simulink model "sensor_fusion_2"  (R2022b)
settings: Solver=FixedStepDiscrete  StartTime=0.0  StopTime=200  RelTol=1e-3  EnableMultiTasking=on
values from neighbouring files (symbols this model uses):
  A = [1.06559801427  0.0478097134081  -0.0142426631232; 0.0478097134081  0.959164863261  -0.0359507847494; -0.0142426631232  -0.0359507847494  0.982079248423]    [run1.mat]    (also in run2.mat)
  b = [2.14306210308 15.720848335 -0.863601368467]    [run1.mat]    (also in run2.mat)
  lut_in_model = [0.705252988187 2.8039042404 3.65243764674 4.31474263379 6.41199264306 8.27776188122 9.84362520272 10.5320461641 11.7803083612 12.6369678359 13.2471074191 13.768187271 ... (20 elements, 1x20)]    [lut5.mat]    (also in run1.mat; run2.mat)
  lut_out_model = [3.92727272727 4.14545454545 4.36363636364 4.58181818182 5.45454545455 6.54545454545 7.63636363636 8.72727272727 9.81818181818 10.9090909091 12 13.0909090909 ... (20 elements, 1x20)]    [lut5.mat]    (also in run1.mat; run2.mat)
undefined symbols (not defined in the file or in its folder): Discrete, ODR, Time
libraries: raspberrypiBasiclib x6, raspberrypiIMUsensorslib x2, matrix_library x1, ctrlSharedLib x1, dspsigops x1, raspberrypiAVlib x1, slpidlib x1
settings Model: Creator=sjohnson  LastModifiedBy=sjohnson
settings SolverCC: PositivePriorityOrder=on
settings OptimizationCC: EnhancedBackFolding=on  PassReuseOutputArgsAs=Individual arguments  ZeroExternalMemoryAtStartup=off  ZeroInternalMemoryAtStartup=off  MaxStackSize=64  OptimizeBlockOrder=speed  DifferentSizesBufferReuse=on  OptimizationCustomize=off  EfficientTunableParamExpr=on
settings DebuggingCC: ParameterTunabilityLossMsg=error
settings HardwareCC: ProdBitPerPointer=32  ProdBitPerSizeT=32  ProdBitPerPtrDiffT=32  ProdLargestAtomicInteger=Long  ProdLargestAtomicFloat=Double  ProdWordSize=32  ProdLongLongMode=on  ProdHWDeviceType=ARM Compatible->ARM Cortex  UseEmbeddedCoderFeatures=off  UseSimulinkCoderFeatures=off
settings RTWCC: Description=Embedded Coder  SystemTargetFile=ert.tlc  HardwareBoard=Raspberry Pi  TLCOptions="-aInlineSetEventsForThisBaseRateFcn=TLC_FALSE -aSuppressMultiTaskScheduler=TLC_FALSE  -aRateBasedStepFcn=0"  TemplateMakefile=ert_default_tmf  Toolchain=GNU GCC Embedded Linux  BuildConfiguration=Faster Runs
settings CodeAppCC: ForceParamTrailComments=on  IgnoreCustomStorageClasses=off  OperatorAnnotations=on  SimulinkDataObjDesc=on  SFDataObjDesc=on  InsertBlockDesc=on
settings ERTTargetCC: SupportNonInlinedSFcns=on  SupportVariableSizeSignals=on  ExtModeTransport=2  ExtModeStaticAlloc=on  ExtModeMexFile=ext_xcp  ExtModeIntrfLevel=Level2 - Open

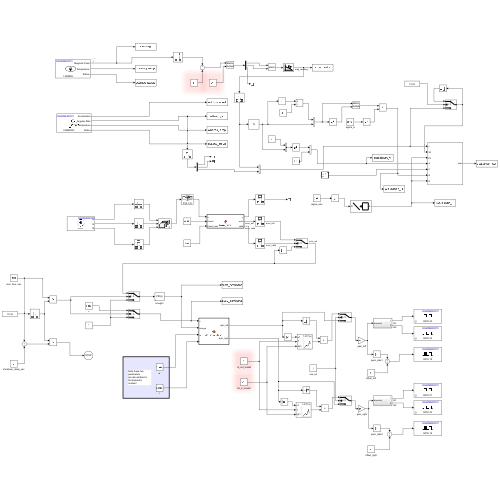
[thumbnail: Simulink's stored preview of the top-level diagram]
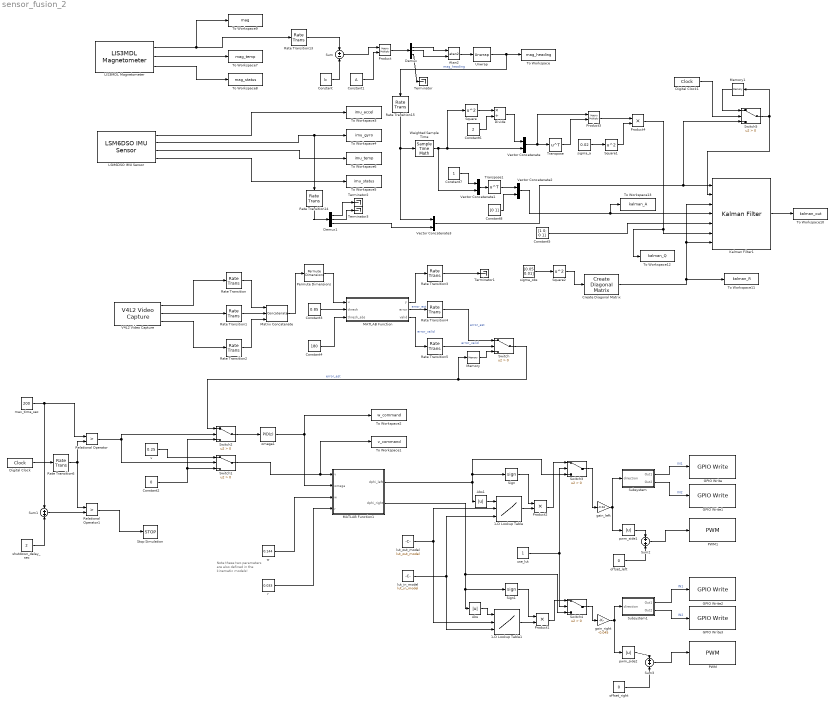
== system sensor_fusion_2 ==
  note: Note these two parameters
      | are also defined in the kinematic
      | models!
  1-D Lookup Table : Lookup_n-D  NumberOfTableDimensions=1  BreakpointsForDimension1Source=Input port  BreakpointsForDimension1=[-5:5]  IndexSearchMethod=Linear search  TableSource=Input port  Table=tanh([-5:5])  InterpMethod=Cubic spline  InternalRulePriority=Speed  RndMeth=Simplest
      settings: InputPortMap=u0,p221,p5
  1-D Lookup Table1 : Lookup_n-D  NumberOfTableDimensions=1  BreakpointsForDimension1Source=Input port  BreakpointsForDimension1=[-5:5]  IndexSearchMethod=Linear search  TableSource=Input port  Table=tanh([-5:5])  InterpMethod=Cubic spline  InternalRulePriority=Speed  RndMeth=Simplest
      settings: InputPortMap=u0,p221,p5
  Abs : Abs  SaturateOnIntegerOverflow=off
  Abs1 : Abs  SaturateOnIntegerOverflow=off
  Atan2 : Trigonometry  Operator=atan2
  Constant : Constant  Value=b  SampleTime=-1
  Constant1 : Constant  Value=A  SampleTime=-1
  Constant2 : Constant  Value=0
  Constant3 : Constant  Value=0.85
  Constant4 : Constant  Value=180
  Constant5 : Constant  Value=[1 0; 0 1]  SampleTime=-1
  Constant6 : Constant  Value=2  SampleTime=-1
  Constant7 : Constant  SampleTime=-1
  Constant8 : Constant  Value=[0 1]  VectorParams1D=off  SampleTime=-1
  Create Diagonal Matrix : matrix_library/Create Diagonal Matrix
      settings: LibrarySourceBlock=|
      | simulink/Matrix
      | Operations/Create Diagonal
      | Matrix
  Demux : Demux  Outputs=3
  Demux1 : Demux  Outputs=3
  Digital Clock : DigitalClock  SampleTime=1/30
  Digital Clock1 : DigitalClock  SampleTime=1/30
  Divide : Product  Inputs=*/
  GPIO Write : raspberrypiBasiclib/GPIO Write  board=Pi 4 Model B  gpio=23  direction=Output  blockPlatform=Raspberry Pi
  GPIO Write1 : raspberrypiBasiclib/GPIO Write  board=Pi 4 Model B  gpio=24  direction=Output  blockPlatform=Raspberry Pi
  GPIO Write2 : raspberrypiBasiclib/GPIO Write  board=Pi 4 Model B  gpio=27  direction=Output  blockPlatform=Raspberry Pi
  GPIO Write3 : raspberrypiBasiclib/GPIO Write  board=Pi 4 Model B  gpio=22  direction=Output  blockPlatform=Raspberry Pi
  Kalman Filter1 : ctrlSharedLib/Kalman Filter  TimeDomain=Discrete-Time  UseCurrentEstimator=on  ModelSource=Input port  ModelSourceVariable=ss(0.95,1,1,0,1)  A=0.95  B=1  C=1  D=0  NumberOfStates=2  NumberOfInputs=1  NumberOfOutputs=2  InitialEstimateSource=Input port  X0=0  P0=10  UseK=off  UseGH=off  NumberOfProcessNoiseInputs=1  G=1  TimeInvariantG=on  H=0  TimeInvariantH=on  Q=0.05  TimeInvariantQ=off  R=[0.0025 0; 0 0.0001]  TimeInvariantR=off  N=0  TimeInvariantN=on  AddInputPort=off  AddEnablePort=off  OutputEstimatedY=off  OutputP=off  Ts=-1
  LIS3MDL Magnetometer : raspberrypiIMUsensorslib/LIS3MDL Magnetometer  I2CModule=1  I2CAddress=0x1E  IsActiveMagnetometer=on  IsActiveTemperature=on  IsStatus=on  SampleTime=1/30  MagnetometerRange=+/- 400 uT  MagnetometerODR=40 Hz
  LSM6DSO IMU Sensor : raspberrypiIMUsensorslib/LSM6DSO IMU Sensor  I2CModule=1  I2CAddress=0x6B  IsActiveAcceleration=on  IsActiveAngularRate=on  IsActiveTemperature=on  IsActiveStatus=on  IsActiveTimeStamp=off  SampleTime=1/30  QueueSizeFactor=3  AccelerometerRange=+/- 2g  AccelerometerODR=52 Hz  AccelSelectCompositeFilter=No filter  AccelLPF2BW=ODR/4  AccelHPFBW=ODR/4  GyroscopeRange=1000 dps  GyroscopeODR=52 Hz  EnableGyroHPF=off  GyroHPFBW=0.016 Hz  EnableGyroLPF=off  GyroLPFBWMode=0
  MATLAB Function : MATLAB Function  TreatAsAtomicUnit=on
  MATLAB Function1 : MATLAB Function  TreatAsAtomicUnit=on
  Matrix Concatenate : Concatenate  NumInputs=3  Mode=Multidimensional array  ConcatenateDimension=3
  Memory : Memory
  Memory1 : Memory  InheritSampleTime=on
  PWM : raspberrypiBasiclib/PWM  board=Pi 4 Model B  Pin_=19  Frequency=40  blockPlatform=Raspberry Pi
  PWM1 : raspberrypiBasiclib/PWM  board=Pi 4 Model B  Pin_=18  Frequency=40  blockPlatform=Raspberry Pi
  Permute Dimensions : PermuteDimensions  Order=[2,1,3]
  Product : Product  Multiplication=Matrix(*)
  Product1 : Product
  Product2 : Product
  Product3 : Product  Multiplication=Matrix(*)
  Product4 : Product
  Rate Transition{,1..6,13} (8 alike) : RateTransition
  Rate Transition14 : RateTransition  OutPortSampleTime=1/30
  Rate Transition15 : RateTransition  OutPortSampleTime=1/30
  Relational Operator : RelationalOperator  Operator=>  OutDataTypeStr=boolean  RndMeth=Simplest  InputSameDT=off
  Relational Operator1 : RelationalOperator  Operator=>  OutDataTypeStr=boolean  RndMeth=Simplest  InputSameDT=off
  Sign : Signum
  Sign1 : Signum
  Square : Math  Operator=square
  Square1 : Math  Operator=square
  Square2 : Math  Operator=square
  Stop Simulation : Stop
  Subsystem : Subsystem
  Subsystem1 : Subsystem
  Sum : Sum  Inputs=+-
  Sum1 : Sum
  Sum2 : Sum
  Sum3 : Sum
  Switch{,1..5} (6 alike) : Switch  Criteria=u2 > Threshold  SaturateOnIntegerOverflow=off  InputSameDT=off
  Terminator{,1..3} (4 alike) : Terminator
  To Workspace : ToWorkspace  VariableName=mag_heading  SaveFormat=Structure With Time  SampleTime=-1
  To Workspace1 : ToWorkspace  VariableName=v_command  SaveFormat=Structure With Time  SampleTime=-1
  To Workspace10 : ToWorkspace  VariableName=kalman_out  SaveFormat=Structure With Time  SampleTime=-1
  To Workspace11 : ToWorkspace  VariableName=kalman_R  SaveFormat=Structure With Time  SampleTime=-1
  To Workspace12 : ToWorkspace  VariableName=kalman_Q  SaveFormat=Structure With Time  SampleTime=-1
  To Workspace13 : ToWorkspace  VariableName=kalman_A  SaveFormat=Structure With Time  SampleTime=-1
  To Workspace2 : ToWorkspace  VariableName=w_command  SaveFormat=Structure With Time  SampleTime=-1
  To Workspace3 : ToWorkspace  VariableName=imu_accel  SaveFormat=Structure With Time  SampleTime=-1
  To Workspace4 : ToWorkspace  VariableName=imu_gyro  SaveFormat=Structure With Time  SampleTime=-1
  To Workspace5 : ToWorkspace  VariableName=imu_status  SaveFormat=Structure With Time  SampleTime=-1
  To Workspace6 : ToWorkspace  VariableName=imu_temp  SaveFormat=Structure With Time  SampleTime=-1
  To Workspace7 : ToWorkspace  VariableName=mag_temp  SaveFormat=Structure With Time  SampleTime=-1
  To Workspace8 : ToWorkspace  VariableName=mag_status  SaveFormat=Structure With Time  SampleTime=-1
  To Workspace9 : ToWorkspace  VariableName=mag  SaveFormat=Structure With Time  SampleTime=-1
  Transpose : Math  Operator=transpose
  Transpose1 : Math  Operator=transpose
  Unwrap : dspsigops/Unwrap  tol=pi  InputProcessing=Columns as channels (frame based)  running=off
  V4L2 Video Capture : raspberrypiAVlib/V4L2 Video Capture  DeviceName=/dev/video0  Resolution=640x480  CustomResolution=[ 320, 240 ]  PixelFormat=RGB  SampleTime=1/30  pixelOrder=planar  simOutput=Colorbars  imSizeSelection=320x240  imSize=[640, 480]  roi=[0, 0, 640, 480]  m_devName='/dev/video0'  blockPlatform=LINUX  HorizontalFlip=off  VerticalFlip=off  Brightness=0.5  Saturation=0.5  Contrast=0.5  Sharpness=0.5  CameraPan=0  CameraTilt=0  CameraZoom=0.5  EnableManualFocus=off  ManualFocus=0.5
  Vector Concatenate : Concatenate  Mode=Multidimensional array
  Vector Concatenate1 : Concatenate
  Vector Concatenate2 : Concatenate  Mode=Multidimensional array
  Vector Concatenate3 : Concatenate  Mode=Multidimensional array
  Weighted Sample Time : SampleTimeMath  TsampMathOp=Ts Only  weightValue=1
  gain_left : Gain  Gain=-0.04
  gain_right : Gain  Gain=-0.045
  lut_in_model : Constant  Value=lut_in_model
  lut_out_model : Constant  Value=lut_out_model
  max_time_sec : Constant  Value=200
  offset_left : Constant  Value=0
  offset_right : Constant  Value=0
  omega1 : slpidlib/PID Controller  Controller=PID  Form=Parallel  TimeDomain=Discrete-time  UseExternalTs=off  SampleTime=-1  IntegratorMethod=Forward Euler  FilterMethod=Forward Euler  ControllerParametersSource=internal  P=-1.5  I=0  UseKiTs=off  D=0  N=100  UseFilter=on  TunerSelectOption=Transfer Function Based (PID Tuner App)  InitialConditionSource=internal  InitialConditionForIntegrator=0  InitialConditionForFilter=0  DifferentiatorICPrevScaledInput=0  ExternalReset=none  TrackingMode=off  Kt=1  LimitOutput=off  SatLimitsSource=internal  UpperSaturationLimit=inf  LowerSaturationLimit=-inf  LinearizeAsGain=off  AntiWindupMode=none  Kb=1  LimitIntegrator=off  UpperIntegratorSaturationLimit=inf  LowerIntegratorSaturationLimit=-inf  POutMin=[]  POutMax=[]  IOutMin=[]  IOutMax=[]  DOutMin=[]  DOutMax=[]  NOutMin=[]  NOutMax=[]  SumOutMin=[]  SumOutMax=[]  SaturationOutMin=[]  SaturationOutMax=[]  PParamMin=[]  PParamMax=[]  IParamMin=[]  IParamMax=[]  DParamMin=[]  DParamMax=[]  NParamMin=[]  NParamMax=[]  KbParamMin=[]  KbParamMax=[]  KtParamMin=[]  KtParamMax=[]  KbOutMin=[]  KbOutMax=[]  KtOutMin=[]  KtOutMax=[]  IntegratorOutMin=[]  IntegratorOutMax=[]  FilterOutMin=[]  FilterOutMax=[]  SumI1OutMin=[]  SumI1OutMax=[]  SumI2OutMin=[]  SumI2OutMax=[]  SumI3OutMin=[]  SumI3OutMax=[]  SumI4OutMin=[]  SumI4OutMax=[]  SumDOutMin=[]  SumDOutMax=[]  DifferentiatorOutMin=[]  DifferentiatorOutMax=[]  FilterDiffOutCoefMin=[]  FilterDiffOutCoefMax=[]  ReciprocalOutMin=[]  ReciprocalOutMax=[]  SumDenOutMin=[]  SumDenOutMax=[]  SumNumOutMin=[]  SumNumOutMax=[]  DivideOutMin=[]  DivideOutMax=[]  UdiffTsProdOutMin=[]  UdiffTsProdOutMax=[]  NTsProdOutMin=[]  NTsProdOutMax=[]  UintegralTsProdOutMin=[]  UintegralTsProdOutMax=[]  UngainTsProdOutMin=[]  UngainTsProdOutMax=[]  ClampingZeroOutDataTypeStr=Inherit: Inherit via back propagation  ClampingZeroOutMin=[]  ClampingZeroOutMax=[]  FilterDenConstantOutDataTypeStr=Inherit: Inherit via back propagation  FilterDenConstantOutMin=[]  FilterDenConstantOutMax=[]  PCopyOutDataTypeStr=Inherit: Inherit via back propagation  PCopyOutMin=[]  PCopyOutMax=[]  NCopyOutDataTypeStr=Inherit: Inherit via back propagation  NCopyOutMin=[]  NCopyOutMax=[]  IntegratorContinuousStateAttributes=''  IntegratorStateMustResolveToSignalObject=off  IntegratorRTWStateStorageClass=Auto  FilterContinuousStateAttributes=''  FilterStateMustResolveToSignalObject=off  FilterRTWStateStorageClass=Auto  ParallelPVariant=InternalParameters  IdealPVariant=Disabled  IVariant=InternalParameters  DVariant=InternalParameters  IntegratorVariant=Discrete  SatVariant=Disabled  AWVariant=Passthrough  PCopyVariant=Disabled  TRVariant=Disabled  FdbkBlocksVariant=Forward  IdealPFdbkVariant=Disabled  SatFdbkVariant=Disabled  DerivativeFilterVariant=ForwardEulerFilter  NVariant=InternalParameters  NCopyVariant=Disabled  FilterICVariant=InternalICsFilter  IntegratorICVariant=InternalICs  ExternalResetVariant=Disabled  TRSumVariant=Passthrough  SumFdbkVariant=Disabled  SumVariant=Sum_PID  TsampFilterVariant=InternalTs  TsampNgainVariant=Passthrough  TsampIntegralVariant=Passthrough  ExternalSaturationOutDataTypeStr=Inherit: Same as second input
      settings: LibrarySourceBlock=simulink/Discrete/Discrete PID Controller
  pwm_side1 : Abs  SaturateOnIntegerOverflow=off
  pwm_side2 : Abs  SaturateOnIntegerOverflow=off
  r : Constant  Value=0.033
  shutdown_delay_sec : Constant  Value=2
  sigma_a : Constant  Value=0.02  SampleTime=-1
  sigma_obs : Constant  Value=[0.05 0.01]  SampleTime=-1
  use_lut : Constant
  v : Constant  Value=0.25
  w : Constant  Value=0.144
  wires:
  LSM6DSO IMU Sensor/3 -> To Workspace6/1
  LIS3MDL Magnetometer/3 -> To Workspace8/1
  LSM6DSO IMU Sensor/1 -> To Workspace3/1
  Constant/1 -> Sum/2
  LIS3MDL Magnetometer/2 -> To Workspace7/1
  Product/1 -> Demux/1
  Demux/2 -> Atan2/2
  Demux/3 -> Terminator/1
  LSM6DSO IMU Sensor/2 -> To Workspace4/1, Rate Transition14/1
  Demux/1 -> Atan2/1
  LSM6DSO IMU Sensor/4 -> To Workspace5/1
  Sum/1 -> Product/1
  Constant1/1 -> Product/2
  Atan2/1 -> Unwrap/1
  LIS3MDL Magnetometer/1 -> To Workspace9/1, Rate Transition13/1
  Unwrap/1 -> Rate Transition15/1, To Workspace/1  "mag_heading"
  gain_left/1 -> pwm_side1/1, Subsystem/1(direction)
  Product1/1 -> Switch4/1
  1-D Lookup Table/1 -> Product2/2
  Rate Transition/1 -> Matrix Concatenate/1
  1-D Lookup Table1/1 -> Product1/2
  Rate Transition6/1 -> Relational Operator1/1, Relational Operator/2
  MATLAB Function/2(error) -> Rate Transition4/1  "error_est"
  Switch/1 -> Switch2/1, Memory/1  "error_est"
  Subsystem/2(Out2) -> GPIO Write1/1  "IN2"
  pwm_side1/1 -> Sum2/1
  Subsystem1/1(Out1) -> GPIO Write2/1  "IN1"
  Rate Transition2/1 -> Matrix Concatenate/3
  MATLAB Function/1(y) -> Rate Transition3/1
  Constant4/1 -> MATLAB Function/3(thresh_abs)
  Rate Transition5/1 -> Switch/2  "error_valid"
  Subsystem/1(Out1) -> GPIO Write/1  "IN1"
  lut_in_model/1 -> 1-D Lookup Table1/3, 1-D Lookup Table/3
  Constant3/1 -> MATLAB Function/2(thresh)
  Sum3/1 -> PWM/1
  Subsystem1/2(Out2) -> GPIO Write3/1  "IN2"
  Constant2/1 -> Switch2/3, Switch1/3
  Memory/1 -> Switch/3
  v/1 -> Switch1/1
  Sum2/1 -> PWM1/1
  Product2/1 -> Switch3/1
  offset_right/1 -> Sum3/2
  Abs1/1 -> 1-D Lookup Table/1
  Sign/1 -> Product2/1
  Switch3/1 -> gain_left/1
  Relational Operator/1 -> Switch1/2, Switch2/2
  Sum1/1 -> Relational Operator1/2
  V4L2 Video Capture/2 -> Rate Transition1/1
  MATLAB Function1/1(dphi_left) -> Switch3/3, Sign/1, Abs1/1
  pwm_side2/1 -> Sum3/1
  Switch4/1 -> gain_right/1
  shutdown_delay_sec/1 -> Sum1/2
  Abs/1 -> 1-D Lookup Table1/1
  Switch2/1 -> omega1/1
  use_lut/1 -> Switch4/2, Switch3/2
  Relational Operator1/1 -> Stop Simulation/1
  Permute Dimensions/1 -> MATLAB Function/1(u)
  omega1/1 -> MATLAB Function1/2(omega), To Workspace2/1
  gain_right/1 -> pwm_side2/1, Subsystem1/1(direction)
  V4L2 Video Capture/3 -> Rate Transition2/1
  Matrix Concatenate/1 -> Permute Dimensions/1
  MATLAB Function1/2(dphi_right) -> Switch4/3, Sign1/1, Abs/1
  w/1 -> MATLAB Function1/3(w)
  MATLAB Function/3(valid) -> Rate Transition5/1  "error_valid"
  Sign1/1 -> Product1/1
  Rate Transition1/1 -> Matrix Concatenate/2
  offset_left/1 -> Sum2/2
  Rate Transition3/1 -> Terminator1/1
  Digital Clock/1 -> Rate Transition6/1
  V4L2 Video Capture/1 -> Rate Transition/1
  max_time_sec/1 -> Relational Operator/1, Sum1/1
  r/1 -> MATLAB Function1/4(r)
  lut_out_model/1 -> 1-D Lookup Table1/2, 1-D Lookup Table/2
  Rate Transition4/1 -> Switch/1  "error_est"
  Switch1/1 -> To Workspace1/1, MATLAB Function1/1(v)
  Weighted Sample Time/1 -> Vector Concatenate1/2, Square/1, Vector Concatenate/2
  Square/1 -> Divide/1
  Constant6/1 -> Divide/2
  Divide/1 -> Vector Concatenate/1
  Vector Concatenate/1 -> Product3/1, Transpose/1
  Transpose/1 -> Product3/2
  sigma_a/1 -> Square1/1
  Product3/1 -> Product4/1
  Square1/1 -> Product4/2
  Constant7/1 -> Vector Concatenate1/1
  Vector Concatenate1/1 -> Transpose1/1
  Transpose1/1 -> Vector Concatenate2/1
  Constant8/1 -> Vector Concatenate2/2
  sigma_obs/1 -> Square2/1
  Square2/1 -> Create Diagonal Matrix/1
  Demux1/3 -> Vector Concatenate3/2
  Demux1/1 -> Terminator2/1
  Demux1/2 -> Terminator3/1
  Digital Clock1/1 -> Switch5/2
  Memory1/1 -> Switch5/1
  Kalman Filter1/1 -> To Workspace10/1
  Vector Concatenate3/1 -> Switch5/3, Kalman Filter1/1
  Vector Concatenate2/1 -> To Workspace13/1, Kalman Filter1/4
  Constant5/1 -> Kalman Filter1/5
  Create Diagonal Matrix/1 -> To Workspace11/1, Kalman Filter1/3, Kalman Filter1/7
  Product4/1 -> To Workspace12/1, Kalman Filter1/6
  Switch5/1 -> Kalman Filter1/2, Memory1/1
  Rate Transition13/1 -> Sum/1
  Rate Transition14/1 -> Demux1/1
  Rate Transition15/1 -> Vector Concatenate3/1, Weighted Sample Time/1

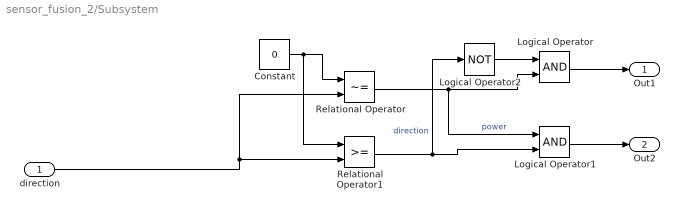
== system sensor_fusion_2/Subsystem ==
  direction : Inport
  Constant : Constant  Value=0
  Logical Operator : Logic  AllPortsSameDT=off  OutDataTypeStr=boolean
  Logical Operator1 : Logic  AllPortsSameDT=off  OutDataTypeStr=boolean
  Logical Operator2 : Logic  Operator=NOT  Inputs=1  AllPortsSameDT=off  OutDataTypeStr=boolean
  Relational Operator : RelationalOperator  Operator=~=  OutDataTypeStr=boolean  RndMeth=Simplest  InputSameDT=off
  Relational Operator1 : RelationalOperator  OutDataTypeStr=boolean  RndMeth=Simplest  InputSameDT=off
  Out1 : Outport
  Out2 : Outport  Port=2
  wires:
  Logical Operator/1 -> Out1/1
  Relational Operator1/1 -> Logical Operator2/1, Logical Operator1/2  "direction"
  Logical Operator1/1 -> Out2/1
  Logical Operator2/1 -> Logical Operator/1
  direction/1 -> Relational Operator/2, Relational Operator1/2
  Constant/1 -> Relational Operator1/1, Relational Operator/1
  Relational Operator/1 -> Logical Operator1/1, Logical Operator/2  "power"

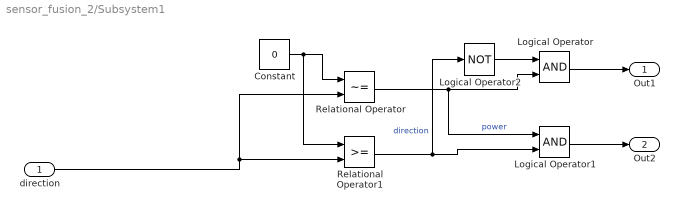
== system sensor_fusion_2/Subsystem1 ==
  direction : Inport
  Constant : Constant  Value=0
  Logical Operator : Logic  AllPortsSameDT=off  OutDataTypeStr=boolean
  Logical Operator1 : Logic  AllPortsSameDT=off  OutDataTypeStr=boolean
  Logical Operator2 : Logic  Operator=NOT  Inputs=1  AllPortsSameDT=off  OutDataTypeStr=boolean
  Relational Operator : RelationalOperator  Operator=~=  OutDataTypeStr=boolean  RndMeth=Simplest  InputSameDT=off
  Relational Operator1 : RelationalOperator  OutDataTypeStr=boolean  RndMeth=Simplest  InputSameDT=off
  Out1 : Outport
  Out2 : Outport  Port=2
  wires:
  Logical Operator/1 -> Out1/1
  Relational Operator1/1 -> Logical Operator2/1, Logical Operator1/2  "direction"
  Logical Operator1/1 -> Out2/1
  Logical Operator2/1 -> Logical Operator/1
  direction/1 -> Relational Operator/2, Relational Operator1/2
  Constant/1 -> Relational Operator1/1, Relational Operator/1
  Relational Operator/1 -> Logical Operator1/1, Logical Operator/2  "power"

== matlab function sensor_fusion_2/MATLAB Function1 ==
  data: v input; dphi_left output; omega input; w input; r input; dphi_right output
function [dphi_left, dphi_right] = diff_drive_xform(v, omega, w, r)

c1 = w/(2*r);
c2 = 2/w;

dphi_left = c1 * ( c2*v - omega );
dphi_right = c1 * ( c2*v + omega );

== matlab function sensor_fusion_2/MATLAB Function ==
  data: u input; y output; error output; valid output; thresh input; thresh_abs input
function [y, error, valid] = image_strip(u, thresh, thresh_abs)
% trim out horizontal slice of image
y = u(325:425, :, :);
dy = double(y);
redness = dy(:,:,1)./vecnorm(dy,1,3) .* dy(:,:,1)>thresh_abs;
y_reduction = max(redness,[],1);
fmin = find(y_reduction>thresh, 1, 'first');
fmax = find(y_reduction>thresh, 1, 'last');
if isempty(fmin) | isempty(fmax)
    valid = 0;
    error = nan;
else
    valid = 1;
    min_value = [find(y_reduction>thresh, 1, 'first')];
    max_value = [find(y_reduction>thresh, 1, 'last')];
    error = ((max_value(1) + min_value(1))/2 - 320)/320;
end
